simulink model "speed_esc_closed_loop"  (R2022b)
settings: Solver=FixedStepDiscrete  StartTime=0.0  StopTime=119.90000000000001  FixedStep=0.10000000000000001  RelTol=1e-3
InitFcn:
  | addpath(fileparts(fileparts(get_param(bdroot,'FileName'))));
model workspace (MAT data in the model file):
  noise_input = [0 0.1 0.2 0.3 0.4 0.5 0.6 0.7 0.8 0.9 1 1.1 ... (2400 elements, 1200x2)]
  private_optimum_input = [0 0.1 0.2 0.3 0.4 0.5 0.6 0.7 0.8 0.9 1 1.1 ... (2400 elements, 1200x2)]
  speed_configuration : object (value not decoded)
  valid_input = [0 0.1 0.2 0.3 0.4 0.5 0.6 0.7 0.8 0.9 1 1.1 ... (2400 elements, 1200x2)]
(part 2 of 2)

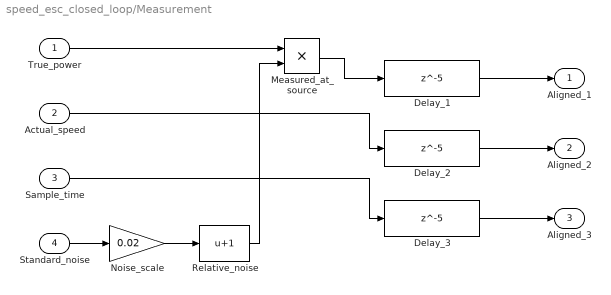
== system speed_esc_closed_loop/Measurement ==
  True_power : Inport
  Actual_speed : Inport  Port=2
  Sample_time : Inport  Port=3
  Standard_noise : Inport  Port=4
  Delay_1 : Delay  DelayLength=5  InitialCondition=1.0247957378670685  SampleTime=0.10000000000000001
  Delay_2 : Delay  DelayLength=5  InitialCondition=10  SampleTime=0.10000000000000001
  Delay_3 : Delay  DelayLength=5  InitialCondition=0  SampleTime=0.10000000000000001
  Measured_at_source : Product
  Noise_scale : Gain  Gain=0.02
  Relative_noise : Bias  Bias=1  SaturateOnIntegerOverflow=off
  Aligned_1 : Outport
  Aligned_2 : Outport  Port=2
  Aligned_3 : Outport  Port=3
  wires:
  Standard_noise/1 -> Noise_scale/1
  Noise_scale/1 -> Relative_noise/1
  True_power/1 -> Measured_at_source/1
  Relative_noise/1 -> Measured_at_source/2
  Measured_at_source/1 -> Delay_1/1
  Delay_1/1 -> Aligned_1/1
  Actual_speed/1 -> Delay_2/1
  Delay_2/1 -> Aligned_2/1
  Sample_time/1 -> Delay_3/1
  Delay_3/1 -> Aligned_3/1

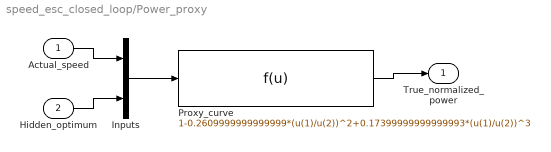
== system speed_esc_closed_loop/Power_proxy ==
  Actual_speed : Inport
  Hidden_optimum : Inport  Port=2
  Inputs : Mux  Inputs=2
  Proxy_curve : Fcn  Expr=1-0.2609999999999999*(u(1)/u(2))^2+0.17399999999999993*(u(1)/u(2))^3
  True_normalized_power : Outport
  wires:
  Actual_speed/1 -> Inputs/1
  Hidden_optimum/1 -> Inputs/2
  Inputs/1 -> Proxy_curve/1
  Proxy_curve/1 -> True_normalized_power/1

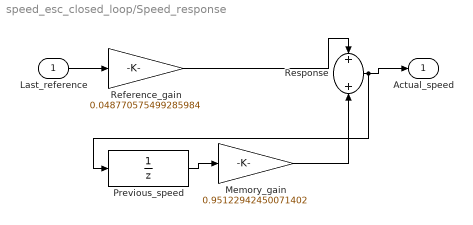
== system speed_esc_closed_loop/Speed_response ==
  Last_reference : Inport
  Memory_gain : Gain  Gain=0.95122942450071402
  Previous_speed : UnitDelay  InitialCondition=10  SampleTime=0.10000000000000001  HasFrameUpgradeWarning=on
  Reference_gain : Gain  Gain=0.048770575499285984
  Response : Sum
  Actual_speed : Outport
  wires:
  Last_reference/1 -> Reference_gain/1
  Reference_gain/1 -> Response/1
  Previous_speed/1 -> Memory_gain/1
  Memory_gain/1 -> Response/2
  Response/1 -> Actual_speed/1, Previous_speed/1

== matlab function speed_esc_closed_loop/Reference_update ==
  data: g input; ref output; ready input; healthy input; now input; center output; dither output; limited output; frozen output
function [ref,center,dither,limited,frozen] = reference_update(g,ready,healthy,now)
%#codegen
persistent s
p=struct('Ts',0.10000000000000001,'lower',0,'upper',20,'amplitude',0.5,'omega',0.5,'gain',8,'hpOmega',0.10000000000000001,'lpOmega',2,'window',126,'minimumSpeedStd',0.025000000000000001,'gradientLimit',1,'centerRate',0.80000000000000004,'referenceRate',1,'maxAge',2,'fixedReference',10,'method',1,'controlMode',2);
if isempty(s), s=speedesc.reference_reset(10,p); end
[ref,s,d]=speedesc.reference_step(s,g,logical(ready),logical(healthy),now,p);
center=d.center; dither=d.dither; limited=double(d.limited); frozen=double(d.frozen);
end

== matlab function speed_esc_closed_loop/Gradient_estimator ==
  data: J input; hp output; paired_v input; sample_time input; now input; valid input; raw output; g output; ready output; healthy output
function [hp,raw,g,ready,healthy] = estimate(J,paired_v,sample_time,now,valid)
%#codegen
persistent s
p=struct('Ts',0.10000000000000001,'lower',0,'upper',20,'amplitude',0.5,'omega',0.5,'gain',8,'hpOmega',0.10000000000000001,'lpOmega',2,'window',126,'minimumSpeedStd',0.025000000000000001,'gradientLimit',1,'centerRate',0.80000000000000004,'referenceRate',1,'maxAge',2,'fixedReference',10,'method',1,'controlMode',2);
if isempty(s), s=speedesc.estimator_reset(p); end
[s,d]=speedesc.estimate_step(s,J,paired_v,sample_time,now,logical(valid),p);
hp=d.highpass; raw=d.rawGradient; g=d.gradient; ready=double(d.ready); healthy=double(d.healthy);
end
